simulink model "simulink"  (R2015a)
settings: Solver=ode4  StartTime=0.0  StopTime=inf  FixedStep=1e-3  RelTol=1e-3
values from neighbouring files (symbols this model uses):
  b_end1 = 0.5*(k_end1*Cyl1.m)^0.5    [m-script.m]
  b_end2 = 0.5*(k_end2*Cyl2.m)^0.5    [m-script.m]
  b_end3 = 0.5*(k_end3*Cyl3.m)^0.5    [m-script.m]
  b_end4 = 0.5*(k_end4*Cyl4.m)^0.5    [m-script.m]
  Cyl1_b = 40000    [m-script.m]
  Cyl1_Fc = 20514    [m-script.m]
  Cyl1_Fs = 22360    [m-script.m]
  Cyl1_K = 20000    [m-script.m]
  Cyl1_vs = 0.8    [m-script.m]
  Cyl2_b = 30000    [m-script.m]
  Cyl2_Fc = 14950    [m-script.m]
  Cyl2_Fs = 16125    [m-script.m]
  Cyl2_K = 20000    [m-script.m]
  Cyl2_vs = 0.8    [m-script.m]
  Cyl3_b = 30000    [m-script.m]
  Cyl3_Fc = 14996    [m-script.m]
  Cyl3_Fs = 16340    [m-script.m]
  Cyl3_K = 20000    [m-script.m]
  Cyl3_vs = 0.8    [m-script.m]
  Cyl4_b = 8500    [m-script.m]
  Cyl4_Fc = 4570    [m-script.m]
  Cyl4_Fs = 4945    [m-script.m]
  Cyl4_K = 20000    [m-script.m]
  Cyl4_vs = 0.8    [m-script.m]
  k_end1 = (pr_Ps*Cyl1.A_A)/v1    [m-script.m]
  k_end2 = (pr_Ps*Cyl2.A_A)/v2    [m-script.m]
  k_end3 = (pr_Ps*Cyl3.A_A)/v3    [m-script.m]
  k_end4 = (pr_Ps*Cyl4.A_A)/v4    [m-script.m]
  pr_Ps = 215e5    (= 21500000)    [m-script.m]
  sampleTime = 0.001    [m-script.m]
  Valve_eta = 0.989    [m-script.m]
  Valve_omega = 40.5    [m-script.m]
undefined symbols (not defined in the file or in its folder): Cyl, Cyl1, Cyl2, Cyl3, Cyl4, Cylinder2, Cylinder3, Cylinder4, Extention1, Extention2, Lift, Link1, Pillar, Pinion, Piston2, Piston3, Piston4, Rack, Tilt, Valve, X, Y, Z
undefined symbols (not defined in the file): Valve1, Valve2, Valve3, Valve4
libraries: sm_lib x72, simulink x32, nesl_utility x20, simulink_extras x3, xpcrtudplib x2, xpcobsoletelib x2
(part 3 of 4)

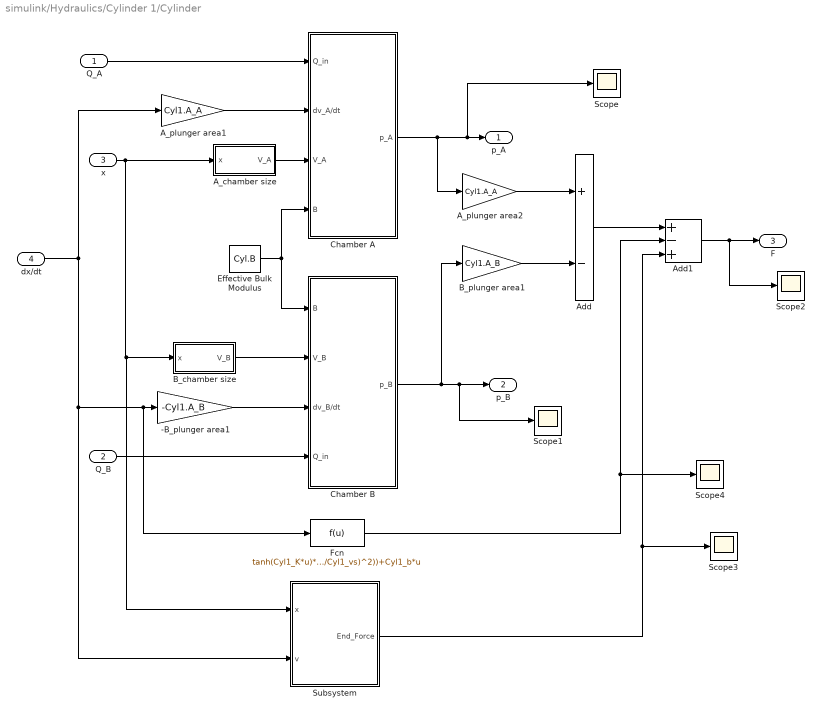
== system simulink/Hydraulics/Cylinder 1/Cylinder ==
  Q_A : Inport
  Q_B : Inport  Port=2
  x : Inport  Port=3
  dx/dt : Inport  Port=4
  -B_plunger area1 : Gain  Gain=-Cyl1.A_B
  A_chamber size : Subsystem
  A_plunger area1 : Gain  Gain=Cyl1.A_A
  A_plunger area2 : Gain  Gain=Cyl1.A_A
  Add : Sum  Inputs=+-
  Add1 : Sum  Inputs=+-+
  B_chamber size : Subsystem
  B_plunger area1 : Gain  Gain=Cyl1.A_B
  Chamber A : Subsystem  mask(Hydraulic){pinitial=Cyl1.pa_init}
      mask prompts: pinitial "Initial pressure [Pa] :"
      mask help: Lumped fluid volume. Pressure is limited greater or equal to zero by saturation block corresponding to a rough model of cavitation.
      mask Help: eval('hydlibdoc(''vol_cav_doc'')')
  Chamber B : Subsystem  mask(Hydraulic){pinitial=Cyl1.pb_init}
      mask prompts: pinitial "Initial pressure [Pa] :"
      mask help: Lumped fluid volume. Pressure is limited greater or equal to zero by saturation block corresponding to a rough model of cavitation.
      mask Help: eval('hydlibdoc(''vol_cav_doc'')')
  Effective Bulk Modulus : Constant  Value=Cyl.B
  Fcn : Fcn  Expr=tanh(Cyl1_K*u)*(Cyl1_Fc+(Cyl1_Fs-Cyl1_Fc)*exp(-1*(u/Cyl1_vs)^2))+Cyl1_b*u
  Scope{,1..4} (5 alike) : Scope
      Scope settings: YMin=4436994.34916  YMax=4451445.07232  SaveName=ScopeData34
      Scope1 settings: YMin=4437551.75654  YMax=4442034.19114  SaveName=ScopeData35
      Scope2 settings: YMin=-2641181.18354  YMax=577446.09906  SaveName=ScopeData5
      Scope3 settings: YMin=-2960719.83587  YMax=328968.87065  SaveName=ScopeData6
      Scope4 settings: YMin=-12307.20024  YMax=12364.555  SaveName=ScopeData7
  Subsystem : Subsystem
  p_A : Outport
  p_B : Outport  Port=2
  F : Outport  Port=3
  wires:
  A_plunger area1/1 -> Chamber A/2(" dv_A/dt")
  dx/dt/1 -> A_plunger area1/1, Subsystem/2(v), Fcn/1, -B_plunger area1/1
  Effective Bulk Modulus/1 -> Chamber A/4(" B"), Chamber B/1(B)
  -B_plunger area1/1 -> Chamber B/3(dv_B/dt)
  A_chamber size/1(V_A) -> Chamber A/3(" V_A")
  Fcn/1 -> Add1/2, Scope4/1
  Q_A/1 -> Chamber A/1(Q_in)
  Chamber A/1(p_A) -> Scope/1, p_A/1, A_plunger area2/1
  Chamber B/1(p_B) -> Scope1/1, p_B/1, B_plunger area1/1
  A_plunger area2/1 -> Add/1
  B_plunger area1/1 -> Add/2
  Add/1 -> Add1/1
  B_chamber size/1(V_B) -> Chamber B/2(V_B)
  Q_B/1 -> Chamber B/4(Q_in)
  Add1/1 -> Scope2/1, F/1
  x/1 -> A_chamber size/1(x), Subsystem/1(x), B_chamber size/1(x)
  Subsystem/1(End_Force) -> Add1/3, Scope3/1

== system simulink/Hydraulics/Cylinder 2/4//3 Valve ==
  p_A : Inport
  p_S : Inport  Port=2
  p_T : Inport  Port=3
  u : Inport  Port=4
  p_B : Inport  Port=5
  Flow paths : Subsystem
  Relative openings : Subsystem
  Valve Dynamics : Subsystem
  Q_P : Outport
  Q_T : Outport  Port=2
  Q_A : Outport  Port=3
  Q_B : Outport  Port=4
  wires:
  Valve Dynamics/1(x) -> Relative openings/1(x)
  Relative openings/1(av_AT) -> Flow paths/5(av_AT)
  Flow paths/4(Q_B) -> Q_B/1
  Flow paths/3(Q_T) -> Q_T/1
  Flow paths/2(Q_P) -> Q_P/1
  Flow paths/1(Q_A) -> Q_A/1
  p_T/1 -> Flow paths/4(p_T)
  p_S/1 -> Flow paths/3(p_S)
  p_B/1 -> Flow paths/2(p_B)
  p_A/1 -> Flow paths/1(p_A)
  Relative openings/2(av_BT) -> Flow paths/6(av_BT)
  Relative openings/3(av_PB) -> Flow paths/7(av_PB)
  Relative openings/4(av_PA) -> Flow paths/8(av_PA)
  u/1 -> Valve Dynamics/1(u)

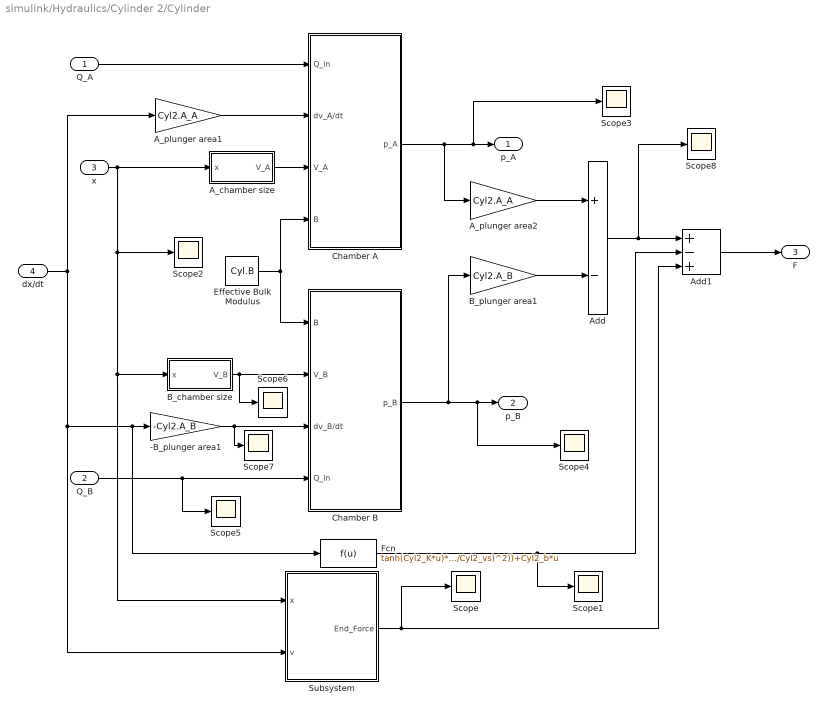
== system simulink/Hydraulics/Cylinder 2/Cylinder ==
  Q_A : Inport
  Q_B : Inport  Port=2
  x : Inport  Port=3
  dx/dt : Inport  Port=4
  -B_plunger area1 : Gain  Gain=-Cyl2.A_B
  A_chamber size : Subsystem
  A_plunger area1 : Gain  Gain=Cyl2.A_A
  A_plunger area2 : Gain  Gain=Cyl2.A_A
  Add : Sum  Inputs=+-
  Add1 : Sum  Inputs=+-+
  B_chamber size : Subsystem
  B_plunger area1 : Gain  Gain=Cyl2.A_B
  Chamber A : Subsystem  mask(Hydraulic){pinitial=Cyl2.pa_init}
      mask prompts: pinitial "Initial pressure [Pa] :"
      mask help: Lumped fluid volume. Pressure is limited greater or equal to zero by saturation block corresponding to a rough model of cavitation.
      mask Help: eval('hydlibdoc(''vol_cav_doc'')')
  Chamber B : Subsystem  mask(Hydraulic){pinitial=Cyl2.pb_init}
      mask prompts: pinitial "Initial pressure [Pa] :"
      mask help: Lumped fluid volume. Pressure is limited greater or equal to zero by saturation block corresponding to a rough model of cavitation.
      mask Help: eval('hydlibdoc(''vol_cav_doc'')')
  Effective Bulk Modulus : Constant  Value=Cyl.B
  Fcn : Fcn  Expr=tanh(Cyl2_K*u)*(Cyl2_Fc+(Cyl2_Fs-Cyl2_Fc)*exp(-1*(u/Cyl2_vs)^2))+Cyl2_b*u
  Scope{,1..8} (9 alike) : Scope
      Scope settings: YMin=-1051842.78204  YMax=116871.42023  SaveName=ScopeData2
      Scope1 settings: YMin=-10637.267  YMax=10226.6678  SaveName=ScopeData4
      Scope2 settings: YMin=0.22817  YMax=0.24759  SaveName=ScopeData5
      Scope3 settings: YMin=10697580.90994  YMax=17121771.81053  SaveName=ScopeData32
      Scope4 settings: YMin=1984662.3633  YMax=2265607.51831  SaveName=ScopeData33
      Scope5 settings: YMin=-0.00000009  YMax=0.00000026
      Scope6 settings: YMin=-0.00041  YMax=0.00539  SaveName=ScopeData2
      Scope7 settings: YMin=-0.00176  YMax=0.00311  SaveName=ScopeData7
      Scope8 settings: YMin=79251.57966  YMax=181198.26244  SaveName=ScopeData2
  Subsystem : Subsystem
  p_A : Outport
  p_B : Outport  Port=2
  F : Outport  Port=3
  wires:
  A_plunger area1/1 -> Chamber A/2(" dv_A/dt")
  dx/dt/1 -> A_plunger area1/1, Fcn/1, -B_plunger area1/1, Subsystem/2(v)
  Effective Bulk Modulus/1 -> Chamber A/4(" B"), Chamber B/1(B)
  x/1 -> A_chamber size/1(x), Scope2/1, Subsystem/1(x), B_chamber size/1(x)
  -B_plunger area1/1 -> Scope7/1, Chamber B/3(dv_B/dt)
  A_chamber size/1(V_A) -> Chamber A/3(" V_A")
  Fcn/1 -> Scope1/1, Add1/2
  Q_A/1 -> Chamber A/1(Q_in)
  Chamber A/1(p_A) -> Scope3/1, p_A/1, A_plunger area2/1
  Chamber B/1(p_B) -> Scope4/1, p_B/1, B_plunger area1/1
  A_plunger area2/1 -> Add/1
  B_plunger area1/1 -> Add/2
  Add/1 -> Scope8/1, Add1/1
  B_chamber size/1(V_B) -> Chamber B/2(V_B), Scope6/1
  Q_B/1 -> Scope5/1, Chamber B/4(Q_in)
  Add1/1 -> F/1
  Subsystem/1(End_Force) -> Scope/1, Add1/3

== system simulink/Hydraulics/Cylinder 3/4//3 Valve ==
  p_A : Inport
  p_S : Inport  Port=2
  p_T : Inport  Port=3
  u : Inport  Port=4
  p_B : Inport  Port=5
  Flow paths : Subsystem
  Relative openings : Subsystem
  Valve Dynamics : Subsystem
  Q_P : Outport
  Q_T : Outport  Port=2
  Q_A : Outport  Port=3
  Q_B : Outport  Port=4
  wires:
  Valve Dynamics/1(x) -> Relative openings/1(x)
  Relative openings/1(av_AT) -> Flow paths/5(av_AT)
  Flow paths/4(Q_B) -> Q_B/1
  Flow paths/3(Q_T) -> Q_T/1
  Flow paths/2(Q_P) -> Q_P/1
  Flow paths/1(Q_A) -> Q_A/1
  p_T/1 -> Flow paths/4(p_T)
  p_S/1 -> Flow paths/3(p_S)
  p_B/1 -> Flow paths/2(p_B)
  p_A/1 -> Flow paths/1(p_A)
  Relative openings/2(av_BT) -> Flow paths/6(av_BT)
  Relative openings/3(av_PB) -> Flow paths/7(av_PB)
  Relative openings/4(av_PA) -> Flow paths/8(av_PA)
  u/1 -> Valve Dynamics/1(u)

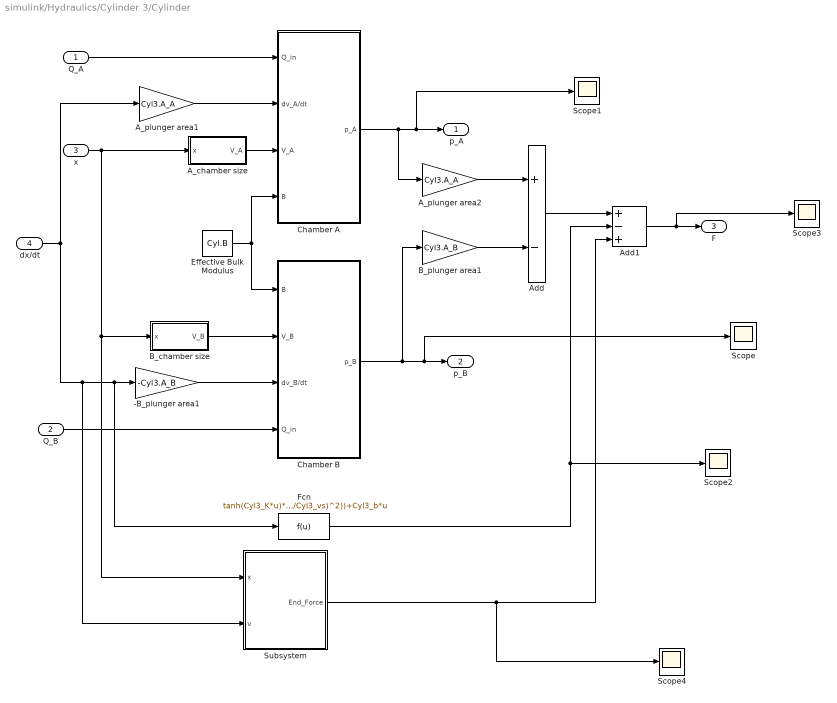
== system simulink/Hydraulics/Cylinder 3/Cylinder ==
  Q_A : Inport
  Q_B : Inport  Port=2
  x : Inport  Port=3
  dx/dt : Inport  Port=4
  -B_plunger area1 : Gain  Gain=-Cyl3.A_B
  A_chamber size : Subsystem
  A_plunger area1 : Gain  Gain=Cyl3.A_A
  A_plunger area2 : Gain  Gain=Cyl3.A_A
  Add : Sum  Inputs=+-
  Add1 : Sum  Inputs=+-+
  B_chamber size : Subsystem
  B_plunger area1 : Gain  Gain=Cyl3.A_B
  Chamber A : Subsystem  mask(Hydraulic){pinitial=Cyl3.pa_init}
      mask prompts: pinitial "Initial pressure [Pa] :"
      mask help: Lumped fluid volume. Pressure is limited greater or equal to zero by saturation block corresponding to a rough model of cavitation.
      mask Help: eval('hydlibdoc(''vol_cav_doc'')')
  Chamber B : Subsystem  mask(Hydraulic){pinitial=Cyl3.pb_init}
      mask prompts: pinitial "Initial pressure [Pa] :"
      mask help: Lumped fluid volume. Pressure is limited greater or equal to zero by saturation block corresponding to a rough model of cavitation.
      mask Help: eval('hydlibdoc(''vol_cav_doc'')')
  Effective Bulk Modulus : Constant  Value=Cyl.B
  Fcn : Fcn  Expr=tanh(Cyl3_K*u)*(Cyl3_Fc+(Cyl3_Fs-Cyl3_Fc)*exp(-1*(u/Cyl3_vs)^2))+Cyl3_b*u
  Scope{,1..4} (5 alike) : Scope
      Scope settings: YMin=-232506.13833  YMax=2092555.24493  SaveName=ScopeData30
      Scope1 settings: YMin=8204020.85918  YMax=9658590.83811  SaveName=ScopeData31
      Scope2 settings: YMin=-10  YMax=10  SaveName=ScopeData2
      Scope3 settings: YMin=-10  YMax=10  SaveName=ScopeData3
      Scope4 settings: YMin=-453635.79942  YMax=50403.97771  SaveName=ScopeData4
  Subsystem : Subsystem
  p_A : Outport
  p_B : Outport  Port=2
  F : Outport  Port=3
  wires:
  A_plunger area1/1 -> Chamber A/2(" dv_A/dt")
  dx/dt/1 -> A_plunger area1/1, Subsystem/2(v), -B_plunger area1/1, Fcn/1
  Effective Bulk Modulus/1 -> Chamber A/4(" B"), Chamber B/1(B)
  x/1 -> A_chamber size/1(x), Subsystem/1(x), B_chamber size/1(x)
  -B_plunger area1/1 -> Chamber B/3(dv_B/dt)
  A_chamber size/1(V_A) -> Chamber A/3(" V_A")
  Fcn/1 -> Scope2/1, Add1/2
  Q_A/1 -> Chamber A/1(Q_in)
  Chamber A/1(p_A) -> Scope1/1, p_A/1, A_plunger area2/1
  Chamber B/1(p_B) -> Scope/1, p_B/1, B_plunger area1/1
  A_plunger area2/1 -> Add/1
  B_plunger area1/1 -> Add/2
  Add/1 -> Add1/1
  B_chamber size/1(V_B) -> Chamber B/2(V_B)
  Q_B/1 -> Chamber B/4(Q_in)
  Subsystem/1(End_Force) -> Scope4/1, Add1/3
  Add1/1 -> Scope3/1, F/1

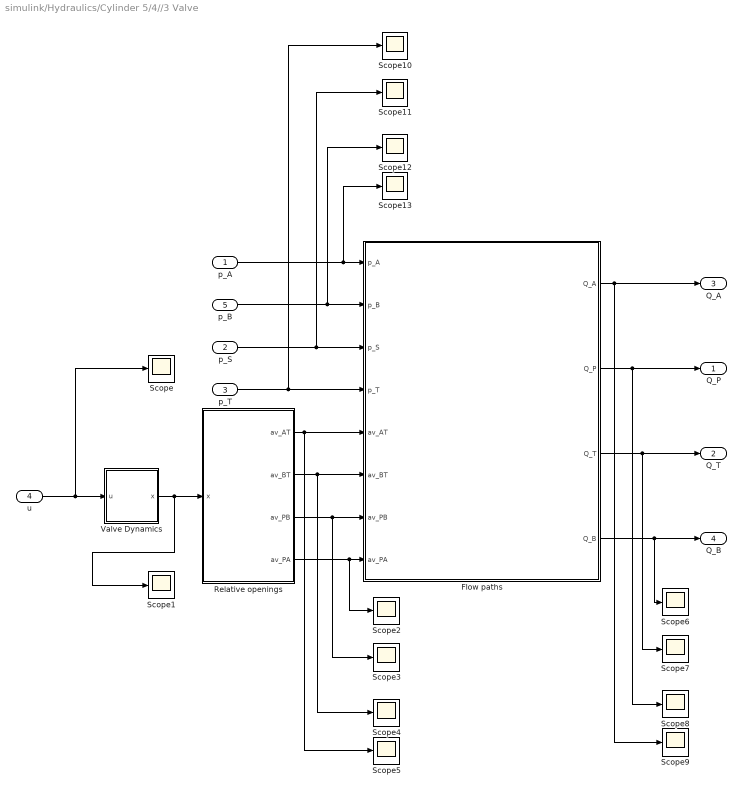
== system simulink/Hydraulics/Cylinder 5/4//3 Valve ==
  p_A : Inport
  p_S : Inport  Port=2
  p_T : Inport  Port=3
  u : Inport  Port=4
  p_B : Inport  Port=5
  Flow paths : Subsystem
  Relative openings : Subsystem
  Scope{,1..13} (14 alike) : Scope
      Scope settings: YMin=-1.00000  YMax=1.00000  SaveName=ScopeData9
      Scope1 settings: YMin=0.1317  YMax=0.45561  SaveName=ScopeData10
      Scope10 settings: YMin=-1.00000  YMax=1.00000  SaveName=ScopeData19
      Scope11 settings: YMin=11500000.00000  YMax=31500000.00000  SaveName=ScopeData20
      Scope12 settings: YMin=-2997924.65507  YMax=26981321.89563  SaveName=ScopeData21
      Scope13 settings: YMin=-2854848.69891  YMax=25693638.29022  SaveName=ScopeData22
      Scope2 settings: YMin=0.00049  YMax=0.00069  SaveName=ScopeData11
      Scope3 settings: YMin=0.00049  YMax=0.00069  SaveName=ScopeData12
      Scope4 settings: YMin=0.00015  YMax=0.00215  SaveName=ScopeData13
      Scope5 settings: YMin=0.00015  YMax=0.00215  SaveName=ScopeData14
      Scope6 settings: YMin=-0.00461  YMax=0.00297  SaveName=ScopeData15
      Scope7 settings: YMin=0.0000081  YMax=0.0000153  SaveName=ScopeData16
      Scope8 settings: YMin=-0.0000093  YMax=-0.000006  SaveName=ScopeData17
      Scope9 settings: YMin=-0.000009  YMax=0.000001  SaveName=ScopeData18
  Valve Dynamics : Subsystem
  Q_P : Outport
  Q_T : Outport  Port=2
  Q_A : Outport  Port=3
  Q_B : Outport  Port=4
  wires:
  u/1 -> Scope/1, Valve Dynamics/1(u)
  Relative openings/3(av_PB) -> Scope3/1, Flow paths/7(av_PB)
  Relative openings/2(av_BT) -> Scope4/1, Flow paths/6(av_BT)
  p_A/1 -> Scope13/1, Flow paths/1(p_A)
  p_B/1 -> Scope12/1, Flow paths/2(p_B)
  p_S/1 -> Scope11/1, Flow paths/3(p_S)
  p_T/1 -> Scope10/1, Flow paths/4(p_T)
  Flow paths/1(Q_A) -> Scope9/1, Q_A/1
  Flow paths/2(Q_P) -> Scope8/1, Q_P/1
  Flow paths/3(Q_T) -> Scope7/1, Q_T/1
  Flow paths/4(Q_B) -> Scope6/1, Q_B/1
  Relative openings/1(av_AT) -> Scope5/1, Flow paths/5(av_AT)
  Valve Dynamics/1(x) -> Scope1/1, Relative openings/1(x)
  Relative openings/4(av_PA) -> Scope2/1, Flow paths/8(av_PA)

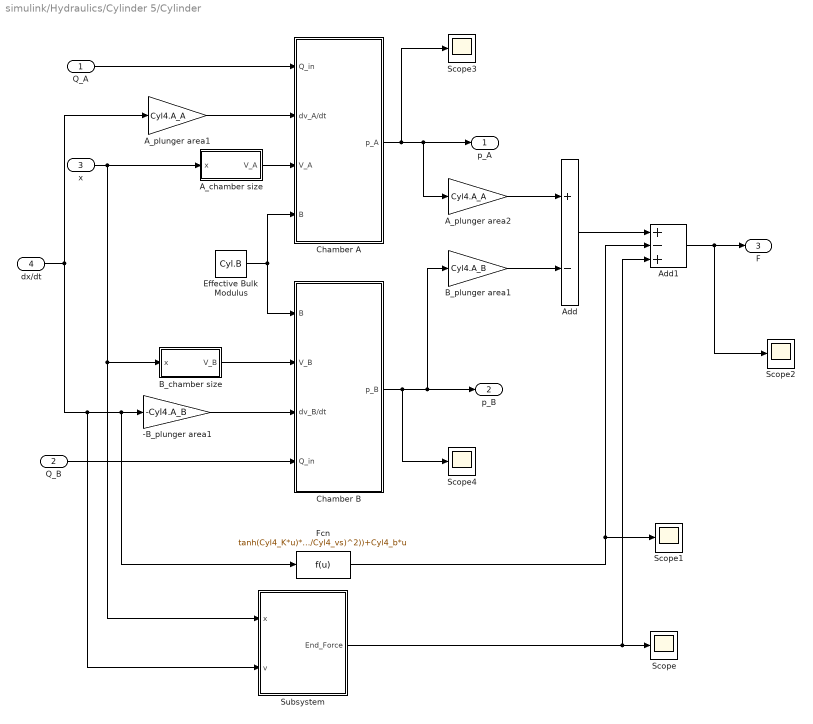
== system simulink/Hydraulics/Cylinder 5/Cylinder ==
  Q_A : Inport
  Q_B : Inport  Port=2
  x : Inport  Port=3
  dx/dt : Inport  Port=4
  -B_plunger area1 : Gain  Gain=-Cyl4.A_B
  A_chamber size : Subsystem
  A_plunger area1 : Gain  Gain=Cyl4.A_A
  A_plunger area2 : Gain  Gain=Cyl4.A_A
  Add : Sum  Inputs=+-
  Add1 : Sum  Inputs=+-+
  B_chamber size : Subsystem
  B_plunger area1 : Gain  Gain=Cyl4.A_B
  Chamber A : Subsystem  mask(Hydraulic){pinitial=Cyl4.pa_init}
      mask prompts: pinitial "Initial pressure [Pa] :"
      mask help: Lumped fluid volume. Pressure is limited greater or equal to zero by saturation block corresponding to a rough model of cavitation.
      mask Help: eval('hydlibdoc(''vol_cav_doc'')')
  Chamber B : Subsystem  mask(Hydraulic){pinitial=Cyl4.pb_init}
      mask prompts: pinitial "Initial pressure [Pa] :"
      mask help: Lumped fluid volume. Pressure is limited greater or equal to zero by saturation block corresponding to a rough model of cavitation.
      mask Help: eval('hydlibdoc(''vol_cav_doc'')')
  Effective Bulk Modulus : Constant  Value=Cyl.B
  Fcn : Fcn  Expr=tanh(Cyl4_K*u)*(Cyl4_Fc+(Cyl4_Fs-Cyl4_Fc)*exp(-1*(u/Cyl4_vs)^2))+Cyl4_b*u
  Scope{,1..4} (5 alike) : Scope
      Scope settings: YMin=-102297.75524  YMax=11366.41725
      Scope1 settings: YMin=-7398.06306  YMax=8052.93154  SaveName=ScopeData2
      Scope2 settings: YMin=-14569.30146  YMax=3367.51691  SaveName=ScopeData3
      Scope3 settings: YMin=2510985.33452  YMax=2517001.5388  SaveName=ScopeData23
      Scope4 settings: YMin=-3100765.75474  YMax=27906891.79262  SaveName=ScopeData24
  Subsystem : Subsystem
  p_A : Outport
  p_B : Outport  Port=2
  F : Outport  Port=3
  wires:
  Subsystem/1(End_Force) -> Scope/1, Add1/3
  Add1/1 -> Scope2/1, F/1
  Q_B/1 -> Chamber B/4(Q_in)
  B_chamber size/1(V_B) -> Chamber B/2(V_B)
  Add/1 -> Add1/1
  B_plunger area1/1 -> Add/2
  A_plunger area2/1 -> Add/1
  Chamber B/1(p_B) -> Scope4/1, B_plunger area1/1, p_B/1
  Chamber A/1(p_A) -> Scope3/1, A_plunger area2/1, p_A/1
  Q_A/1 -> Chamber A/1(Q_in)
  Fcn/1 -> Scope1/1, Add1/2
  A_chamber size/1(V_A) -> Chamber A/3(" V_A")
  -B_plunger area1/1 -> Chamber B/3(dv_B/dt)
  x/1 -> B_chamber size/1(x), Subsystem/1(x), A_chamber size/1(x)
  Effective Bulk Modulus/1 -> Chamber B/1(B), Chamber A/4(" B")
  dx/dt/1 -> Fcn/1, -B_plunger area1/1, Subsystem/2(v), A_plunger area1/1
  A_plunger area1/1 -> Chamber A/2(" dv_A/dt")

== system simulink/Hydraulics/Cylinder 1/4//3 Valve/Flow paths ==
  p_A : Inport
  p_B : Inport  Port=2
  p_S : Inport  Port=3
  p_T : Inport  Port=4
  av_AT : Inport  Port=5
  av_BT : Inport  Port=6
  av_PB : Inport  Port=7
  av_PA : Inport  Port=8
  Orifice AT : Subsystem  mask(Hydraulic){QN=Valve1.QN.AT, dpN=Valve1.dpN, ptr=Valve1.ptr}
      mask prompts: QN "Nominal Flow [m^3/s] :"; dpN "Nominal Pressure Difference [Pa] :"; ptr "Transition Pressure [Pa] :"
      mask help:
      | Implements numerically robust turbulent flow
      | equation. Polynomial flow equation is used
      | when abs(dp) < Transition Pressure.
      mask init:
      | K = QN/(sqrt(dpN));
      mask Help: eval('hydlibdoc(''orificedoc'')')
  Orifice BT : Subsystem  mask(Hydraulic){QN=Valve1.QN.BT, dpN=Valve1.dpN, ptr=Valve1.ptr}
      mask prompts: QN "Nominal Flow [m^3/s] :"; dpN "Nominal Pressure Difference [Pa] :"; ptr "Transition Pressure [Pa] :"
      mask help:
      | Implements numerically robust turbulent flow
      | equation. Polynomial flow equation is used
      | when abs(dp) < Transition Pressure.
      mask init:
      | K = QN/(sqrt(dpN));
      mask Help: eval('hydlibdoc(''orificedoc'')')
  Orifice PA : Subsystem  mask(Hydraulic){QN=Valve1.QN.PA, dpN=Valve1.dpN, ptr=Valve1.ptr}
      mask prompts: QN "Nominal Flow [m^3/s] :"; dpN "Nominal Pressure Difference [Pa] :"; ptr "Transition Pressure [Pa] :"
      mask help:
      | Implements numerically robust turbulent flow
      | equation. Polynomial flow equation is used
      | when abs(dp) < Transition Pressure.
      mask init:
      | K = QN/(sqrt(dpN));
      mask Help: eval('hydlibdoc(''orificedoc'')')
  Orifice PB : Subsystem  mask(Hydraulic){QN=Valve1.QN.PB, dpN=Valve1.dpN, ptr=Valve1.ptr}
      mask prompts: QN "Nominal Flow [m^3/s] :"; dpN "Nominal Pressure Difference [Pa] :"; ptr "Transition Pressure [Pa] :"
      mask help:
      | Implements numerically robust turbulent flow
      | equation. Polynomial flow equation is used
      | when abs(dp) < Transition Pressure.
      mask init:
      | K = QN/(sqrt(dpN));
      mask Help: eval('hydlibdoc(''orificedoc'')')
  Sum{,1..3} (4 alike) : Sum  Inputs=|++
  Q_A : Outport
  Q_P : Outport  Port=2
  Q_T : Outport  Port=3
  Q_B : Outport  Port=4
  wires:
  p_A/1 -> Orifice AT/1(p_A), Orifice PA/2(p_A)
  p_T/1 -> Orifice BT/1(p_T), Orifice AT/2(p_T)
  av_BT/1 -> Orifice BT/3(u)
  av_PA/1 -> Orifice PA/3(u)
  p_B/1 -> Orifice PB/1(p_B), Orifice BT/2(p_B)
  av_PB/1 -> Orifice PB/3(u)
  p_S/1 -> Orifice PB/2(p_P), Orifice PA/1(p_P)
  av_AT/1 -> Orifice AT/3(u)
  Orifice PA/2(Q_A) -> Sum/1
  Orifice AT/1(Q_A) -> Sum/2
  Orifice AT/2(Q_T) -> Sum3/1
  Orifice BT/1(Q_T) -> Sum3/2
  Orifice BT/2(Q_B) -> Sum2/1
  Orifice PB/1(Q_B) -> Sum2/2
  Orifice PA/1(Q_P) -> Sum1/1
  Orifice PB/2(Q_P) -> Sum1/2
  Sum/1 -> Q_A/1
  Sum1/1 -> Q_P/1
  Sum3/1 -> Q_T/1
  Sum2/1 -> Q_B/1

== system simulink/Hydraulics/Cylinder 1/4//3 Valve/Relative openings ==
  x : Inport
  Lookup Table AT : Lookup_n-D  NumberOfTableDimensions=1  BreakpointsForDimension1=Valve.lookupspoolAT  Table=Valve.lookupopenAT  InternalRulePriority=Speed  RndMeth=Simplest  InputSameDT=on
  Lookup Table BT : Lookup_n-D  NumberOfTableDimensions=1  BreakpointsForDimension1=Valve.lookupspoolBT  Table=Valve.lookupopenBT  InternalRulePriority=Speed  RndMeth=Simplest  InputSameDT=on
  Lookup Table PA : Lookup_n-D  NumberOfTableDimensions=1  BreakpointsForDimension1=Valve.lookupspoolPA  Table=Valve.lookupopenPA  InternalRulePriority=Speed  RndMeth=Simplest  InputSameDT=on
  Lookup Table PB : Lookup_n-D  NumberOfTableDimensions=1  BreakpointsForDimension1=Valve.lookupspoolPB  Table=Valve.lookupopenPB  InternalRulePriority=Speed  RndMeth=Simplest  InputSameDT=on
  av_AT : Outport
  av_BT : Outport  Port=2
  av_PB : Outport  Port=3
  av_PA : Outport  Port=4
  wires:
  x/1 -> Lookup Table AT/1, Lookup Table PB/1, Lookup Table BT/1, Lookup Table PA/1
  Lookup Table AT/1 -> av_AT/1
  Lookup Table PA/1 -> av_PA/1
  Lookup Table BT/1 -> av_BT/1
  Lookup Table PB/1 -> av_PB/1

== system simulink/Hydraulics/Cylinder 1/4//3 Valve/Valve Dynamics ==
  u : Inport
  Saturation1 : Saturate  UpperLimit=1  LowerLimit=-1
  Transfer Fcn1 : TransferFcn  Numerator=[(Valve_omega)^2]  Denominator=[1 2*Valve_eta*Valve_omega (Valve_omega)^2]
  Transport Delay1 : TransportDelay  DelayTime=Valve.secondorder_delay
  x : Outport
  wires:
  Transfer Fcn1/1 -> Saturation1/1
  u/1 -> Transport Delay1/1
  Saturation1/1 -> x/1
  Transport Delay1/1 -> Transfer Fcn1/1

== system simulink/Hydraulics/Cylinder 1/Cylinder/A_chamber size ==
  x : Inport
  A_Dead Vol : Constant  Value=Cyl.V0A
  A_plunger area : Gain  Gain=Cyl1.A_A
  Add1 : Sum
  V_A : Outport
  wires:
  A_Dead Vol/1 -> Add1/2
  A_plunger area/1 -> Add1/1
  x/1 -> A_plunger area/1
  Add1/1 -> V_A/1

== system simulink/Hydraulics/Cylinder 1/Cylinder/B_chamber size ==
  x : Inport
  Add2 : Sum  Inputs=-+
  Add4 : Sum
  B_Dead Vol : Constant  Value=Cyl.V0B
  B_plunger area : Gain  Gain=Cyl1.A_B
  Cyl_stroke : Constant  Value=Cyl1.xmax
  V_B : Outport
  wires:
  Add4/1 -> V_B/1
  B_Dead Vol/1 -> Add4/2
  B_plunger area/1 -> Add4/1
  Add2/1 -> B_plunger area/1
  x/1 -> Add2/1
  Cyl_stroke/1 -> Add2/2

== system simulink/Hydraulics/Cylinder 1/Cylinder/Chamber A ==
  Q_in : Inport
  " dv_A/dt" : Inport  Port=2
  " V_A" : Inport  Port=3
  " B" : Inport  Port=4
  Integrator : Integrator  InitialCondition=pinitial  AbsoluteTolerance=10
  Product : Product  Inputs=*/*  SaturateOnIntegerOverflow=on  InputSameDT=on  OutDataTypeStr=Inherit: Same as first input
  Saturation : Saturate  UpperLimit=inf  LowerLimit=0
  Sum : Sum  Inputs=+-  SaturateOnIntegerOverflow=on  InputSameDT=on  OutDataTypeStr=Inherit: Same as first input
  p_A : Outport
  wires:
  Sum/1 -> Product/1
  Q_in/1 -> Sum/1
  " B"/1 -> Product/3
  Saturation/1 -> p_A/1
  Integrator/1 -> Saturation/1
  Product/1 -> Integrator/1
  " dv_A/dt"/1 -> Sum/2
  " V_A"/1 -> Product/2

== system simulink/Hydraulics/Cylinder 1/Cylinder/Chamber B ==
  B : Inport
  V_B : Inport  Port=2
  dv_B/dt : Inport  Port=3
  Q_in : Inport  Port=4
  Integrator : Integrator  InitialCondition=pinitial  AbsoluteTolerance=10
  Product : Product  Inputs=*/*  SaturateOnIntegerOverflow=on  InputSameDT=on  OutDataTypeStr=Inherit: Same as first input
  Saturation : Saturate  UpperLimit=inf  LowerLimit=0
  Sum : Sum  Inputs=+-  SaturateOnIntegerOverflow=on  InputSameDT=on  OutDataTypeStr=Inherit: Same as first input
  p_B : Outport
  wires:
  Product/1 -> Integrator/1
  Integrator/1 -> Saturation/1
  Saturation/1 -> p_B/1
  B/1 -> Product/3
  Q_in/1 -> Sum/1
  Sum/1 -> Product/1
  dv_B/dt/1 -> Sum/2
  V_B/1 -> Product/2

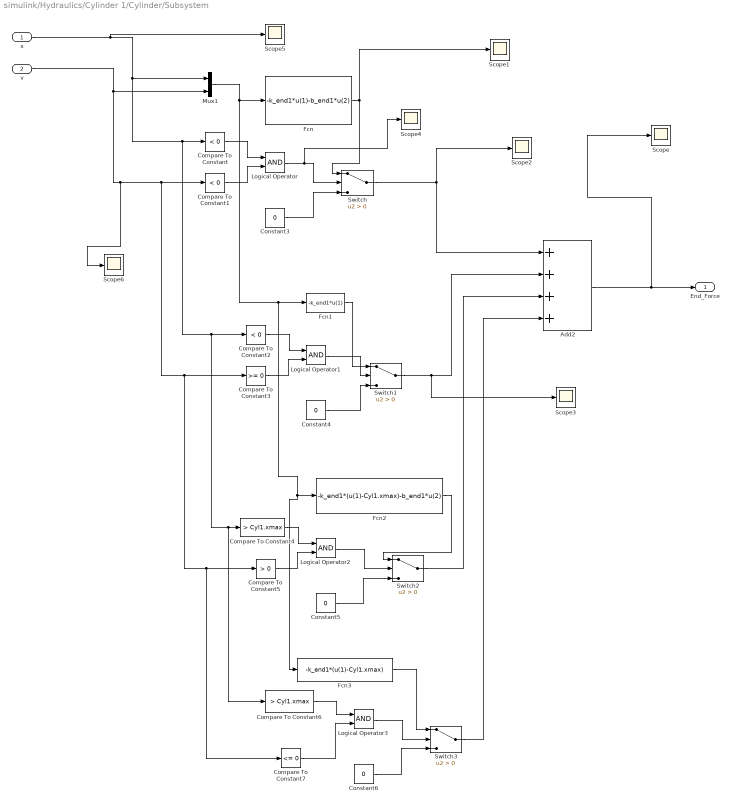
== system simulink/Hydraulics/Cylinder 1/Cylinder/Subsystem ==
  x : Inport
  v : Inport  Port=2
  Add2 : Sum  Inputs=++++
  Compare To Constant : simulink/Logic and Bit Operations/Compare To Constant  relop=<  const=0  OutDataTypeStr=boolean
  Compare To Constant1 : simulink/Logic and Bit Operations/Compare To Constant  relop=<  const=0  OutDataTypeStr=boolean
  Compare To Constant2 : simulink/Logic and Bit Operations/Compare To Constant  relop=<  const=0  OutDataTypeStr=boolean
  Compare To Constant3 : simulink/Logic and Bit Operations/Compare To Constant  relop=>=  const=0  OutDataTypeStr=boolean
  Compare To Constant4 : simulink/Logic and Bit Operations/Compare To Constant  relop=>  const=Cyl1.xmax  OutDataTypeStr=boolean
  Compare To Constant5 : simulink/Logic and Bit Operations/Compare To Constant  relop=>  const=0  OutDataTypeStr=boolean
  Compare To Constant6 : simulink/Logic and Bit Operations/Compare To Constant  relop=>  const=Cyl1.xmax  OutDataTypeStr=boolean
  Compare To Constant7 : simulink/Logic and Bit Operations/Compare To Constant  relop=<=  const=0  OutDataTypeStr=boolean
  Constant{3..6} (4 alike) : Constant  Value=0
  Fcn : Fcn  Expr=-k_end1*u(1)-b_end1*u(2)
  Fcn1 : Fcn  Expr=-k_end1*u(1)
  Fcn2 : Fcn  Expr=-k_end1*(u(1)-Cyl1.xmax)-b_end1*u(2)
  Fcn3 : Fcn  Expr=-k_end1*(u(1)-Cyl1.xmax)
  Logical Operator{,1..3} (4 alike) : Logic  AllPortsSameDT=off  OutDataTypeStr=boolean
  Mux1 : Mux  Inputs=2
  Scope{,1..6} (7 alike) : Scope
      Scope settings: YMin=-1.00000  YMax=1.00000  SaveName=ScopeData7
      Scope1 settings: YMin=-1321864731.63954  YMax=-746398119.03494  SaveName=ScopeData8
      Scope2 settings: YMin=-1.00000  YMax=1.00000  SaveName=ScopeData9
      Scope3 settings: YMin=-1626189.56555  YMax=14635706.08996  SaveName=ScopeData10
      Scope4 settings: YMin=-1.00000  YMax=1.00000  SaveName=ScopeData11
      Scope5 settings: YMin=0.45891  YMax=0.49078  SaveName=ScopeData12
      Scope6 settings: YMin=-0.00619  YMax=0.05469  SaveName=ScopeData13
  Switch{,1..3} (4 alike) : Switch  Criteria=u2 > Threshold
  End_Force : Outport
  wires:
  Compare To Constant3/1 -> Logical Operator1/2
  Fcn1/1 -> Switch1/1
  Compare To Constant4/1 -> Logical Operator2/1
  Compare To Constant/1 -> Logical Operator/1
  Constant3/1 -> Switch/3
  Logical Operator/1 -> Scope4/1, Switch/2
  Fcn/1 -> Switch/1, Scope1/1
  Logical Operator1/1 -> Switch1/2
  Constant4/1 -> Switch1/3
  Constant5/1 -> Switch2/3
  Compare To Constant1/1 -> Logical Operator/2
  Compare To Constant2/1 -> Logical Operator1/1
  Switch3/1 -> Add2/4
  Mux1/1 -> Fcn/1, Fcn3/1, Fcn2/1, Fcn1/1
  Add2/1 -> Scope/1, End_Force/1
  Switch1/1 -> Scope3/1, Add2/2
  Compare To Constant7/1 -> Logical Operator3/2
  Logical Operator2/1 -> Switch2/2
  Switch/1 -> Scope2/1, Add2/1
  Compare To Constant6/1 -> Logical Operator3/1
  Switch2/1 -> Add2/3
  Constant6/1 -> Switch3/3
  Compare To Constant5/1 -> Logical Operator2/2
  Fcn3/1 -> Switch3/1
  Logical Operator3/1 -> Switch3/2
  Fcn2/1 -> Switch2/1
  v/1 -> Scope6/1, Compare To Constant7/1, Compare To Constant5/1, Compare To Constant3/1, Compare To Constant1/1, Mux1/2
  x/1 -> Scope5/1, Mux1/1, Compare To Constant4/1, Compare To Constant6/1, Compare To Constant2/1, Compare To Constant/1

== system simulink/Hydraulics/Cylinder 2/4//3 Valve/Flow paths ==
  p_A : Inport
  p_B : Inport  Port=2
  p_S : Inport  Port=3
  p_T : Inport  Port=4
  av_AT : Inport  Port=5
  av_BT : Inport  Port=6
  av_PB : Inport  Port=7
  av_PA : Inport  Port=8
  Orifice AT : Subsystem  mask(Hydraulic){QN=Valve2.QN.AT, dpN=Valve2.dpN, ptr=Valve2.ptr}
      mask prompts: QN "Nominal Flow [m^3/s] :"; dpN "Nominal Pressure Difference [Pa] :"; ptr "Transition Pressure [Pa] :"
      mask help:
      | Implements numerically robust turbulent flow
      | equation. Polynomial flow equation is used
      | when abs(dp) < Transition Pressure.
      mask init:
      | K = QN/(sqrt(dpN));
      mask Help: eval('hydlibdoc(''orificedoc'')')
  Orifice BT : Subsystem  mask(Hydraulic){QN=Valve2.QN.BT, dpN=Valve2.dpN, ptr=Valve2.ptr}
      mask prompts: QN "Nominal Flow [m^3/s] :"; dpN "Nominal Pressure Difference [Pa] :"; ptr "Transition Pressure [Pa] :"
      mask help:
      | Implements numerically robust turbulent flow
      | equation. Polynomial flow equation is used
      | when abs(dp) < Transition Pressure.
      mask init:
      | K = QN/(sqrt(dpN));
      mask Help: eval('hydlibdoc(''orificedoc'')')
  Orifice PA : Subsystem  mask(Hydraulic){QN=Valve2.QN.PA, dpN=Valve2.dpN, ptr=Valve2.ptr}
      mask prompts: QN "Nominal Flow [m^3/s] :"; dpN "Nominal Pressure Difference [Pa] :"; ptr "Transition Pressure [Pa] :"
      mask help:
      | Implements numerically robust turbulent flow
      | equation. Polynomial flow equation is used
      | when abs(dp) < Transition Pressure.
      mask init:
      | K = QN/(sqrt(dpN));
      mask Help: eval('hydlibdoc(''orificedoc'')')
  Orifice PB : Subsystem  mask(Hydraulic){QN=Valve2.QN.PB, dpN=Valve2.dpN, ptr=Valve2.ptr}
      mask prompts: QN "Nominal Flow [m^3/s] :"; dpN "Nominal Pressure Difference [Pa] :"; ptr "Transition Pressure [Pa] :"
      mask help:
      | Implements numerically robust turbulent flow
      | equation. Polynomial flow equation is used
      | when abs(dp) < Transition Pressure.
      mask init:
      | K = QN/(sqrt(dpN));
      mask Help: eval('hydlibdoc(''orificedoc'')')
  Scope : Scope
      settings: YMin=-0.00424  YMax=0.00506  SaveName=ScopeData3
  Sum{,1..3} (4 alike) : Sum  Inputs=|++
  Q_A : Outport
  Q_P : Outport  Port=2
  Q_T : Outport  Port=3
  Q_B : Outport  Port=4
  wires:
  p_A/1 -> Orifice AT/1(p_A), Orifice PA/2(p_A)
  p_T/1 -> Orifice BT/1(p_T), Orifice AT/2(p_T)
  av_BT/1 -> Orifice BT/3(u)
  av_PA/1 -> Orifice PA/3(u)
  p_B/1 -> Orifice PB/1(p_B), Orifice BT/2(p_B)
  av_PB/1 -> Orifice PB/3(u)
  p_S/1 -> Orifice PB/2(p_P), Orifice PA/1(p_P)
  av_AT/1 -> Orifice AT/3(u)
  Orifice PA/2(Q_A) -> Sum/1
  Orifice AT/1(Q_A) -> Sum/2
  Orifice AT/2(Q_T) -> Sum3/1
  Orifice BT/1(Q_T) -> Sum3/2
  Orifice BT/2(Q_B) -> Sum2/1
  Orifice PB/1(Q_B) -> Sum2/2
  Orifice PA/1(Q_P) -> Sum1/1
  Orifice PB/2(Q_P) -> Sum1/2
  Sum/1 -> Q_A/1
  Sum1/1 -> Q_P/1
  Sum3/1 -> Q_T/1
  Sum2/1 -> Scope/1, Q_B/1

== system simulink/Hydraulics/Cylinder 2/4//3 Valve/Relative openings ==
  x : Inport
  Lookup Table AT : Lookup_n-D  NumberOfTableDimensions=1  BreakpointsForDimension1=Valve.lookupspoolAT  Table=Valve.lookupopenAT  InternalRulePriority=Speed  RndMeth=Simplest  InputSameDT=on
  Lookup Table BT : Lookup_n-D  NumberOfTableDimensions=1  BreakpointsForDimension1=Valve.lookupspoolBT  Table=Valve.lookupopenBT  InternalRulePriority=Speed  RndMeth=Simplest  InputSameDT=on
  Lookup Table PA : Lookup_n-D  NumberOfTableDimensions=1  BreakpointsForDimension1=Valve.lookupspoolPA  Table=Valve.lookupopenPA  InternalRulePriority=Speed  RndMeth=Simplest  InputSameDT=on
  Lookup Table PB : Lookup_n-D  NumberOfTableDimensions=1  BreakpointsForDimension1=Valve.lookupspoolPB  Table=Valve.lookupopenPB  InternalRulePriority=Speed  RndMeth=Simplest  InputSameDT=on
  av_AT : Outport
  av_BT : Outport  Port=2
  av_PB : Outport  Port=3
  av_PA : Outport  Port=4
  wires:
  x/1 -> Lookup Table AT/1, Lookup Table PB/1, Lookup Table BT/1, Lookup Table PA/1
  Lookup Table AT/1 -> av_AT/1
  Lookup Table PA/1 -> av_PA/1
  Lookup Table BT/1 -> av_BT/1
  Lookup Table PB/1 -> av_PB/1

== system simulink/Hydraulics/Cylinder 2/4//3 Valve/Valve Dynamics ==
  u : Inport
  Saturation1 : Saturate  UpperLimit=1  LowerLimit=-1
  Transfer Fcn1 : TransferFcn  Numerator=[(Valve_omega)^2]  Denominator=[1 2*Valve_eta*Valve_omega (Valve_omega)^2]
  Transport Delay1 : TransportDelay  DelayTime=Valve.secondorder_delay
  x : Outport
  wires:
  Transfer Fcn1/1 -> Saturation1/1
  u/1 -> Transport Delay1/1
  Saturation1/1 -> x/1
  Transport Delay1/1 -> Transfer Fcn1/1

== system simulink/Hydraulics/Cylinder 2/Cylinder/A_chamber size ==
  x : Inport
  A_Dead Vol : Constant  Value=Cyl.V0A
  A_plunger area : Gain  Gain=Cyl2.A_A
  Add1 : Sum
  V_A : Outport
  wires:
  A_Dead Vol/1 -> Add1/2
  A_plunger area/1 -> Add1/1
  x/1 -> A_plunger area/1
  Add1/1 -> V_A/1

== system simulink/Hydraulics/Cylinder 2/Cylinder/B_chamber size ==
  x : Inport
  Add2 : Sum  Inputs=-+
  Add4 : Sum
  B_Dead Vol : Constant  Value=Cyl.V0B
  B_plunger area : Gain  Gain=Cyl2.A_B
  Cyl_stroke : Constant  Value=Cyl2.xmax
  V_B : Outport
  wires:
  Add4/1 -> V_B/1
  B_Dead Vol/1 -> Add4/2
  B_plunger area/1 -> Add4/1
  Add2/1 -> B_plunger area/1
  x/1 -> Add2/1
  Cyl_stroke/1 -> Add2/2

== system simulink/Hydraulics/Cylinder 2/Cylinder/Chamber A ==
  Q_in : Inport
  " dv_A/dt" : Inport  Port=2
  " V_A" : Inport  Port=3
  " B" : Inport  Port=4
  Integrator : Integrator  InitialCondition=pinitial  AbsoluteTolerance=10
  Product : Product  Inputs=*/*  SaturateOnIntegerOverflow=on  InputSameDT=on  OutDataTypeStr=Inherit: Same as first input
  Saturation : Saturate  UpperLimit=inf  LowerLimit=0
  Sum : Sum  Inputs=+-  SaturateOnIntegerOverflow=on  InputSameDT=on  OutDataTypeStr=Inherit: Same as first input
  p_A : Outport
  wires:
  Sum/1 -> Product/1
  Q_in/1 -> Sum/1
  " B"/1 -> Product/3
  Saturation/1 -> p_A/1
  Integrator/1 -> Saturation/1
  Product/1 -> Integrator/1
  " dv_A/dt"/1 -> Sum/2
  " V_A"/1 -> Product/2

== system simulink/Hydraulics/Cylinder 2/Cylinder/Chamber B ==
  B : Inport
  V_B : Inport  Port=2
  dv_B/dt : Inport  Port=3
  Q_in : Inport  Port=4
  Integrator : Integrator  InitialCondition=pinitial  AbsoluteTolerance=10
  Product : Product  Inputs=*/*  SaturateOnIntegerOverflow=on  InputSameDT=on  OutDataTypeStr=Inherit: Same as first input
  Saturation : Saturate  UpperLimit=inf  LowerLimit=0
  Sum : Sum  Inputs=+-  SaturateOnIntegerOverflow=on  InputSameDT=on  OutDataTypeStr=Inherit: Same as first input
  p_B : Outport
  wires:
  Product/1 -> Integrator/1
  Integrator/1 -> Saturation/1
  Saturation/1 -> p_B/1
  B/1 -> Product/3
  Q_in/1 -> Sum/1
  Sum/1 -> Product/1
  dv_B/dt/1 -> Sum/2
  V_B/1 -> Product/2

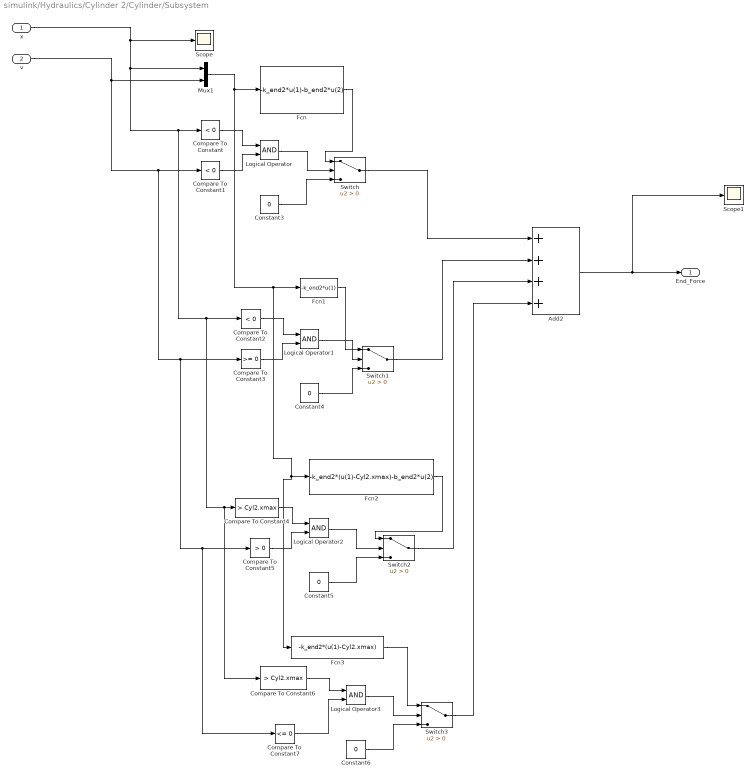
== system simulink/Hydraulics/Cylinder 2/Cylinder/Subsystem ==
  x : Inport
  v : Inport  Port=2
  Add2 : Sum  Inputs=++++
  Compare To Constant : simulink/Logic and Bit Operations/Compare To Constant  relop=<  const=0  OutDataTypeStr=boolean
  Compare To Constant1 : simulink/Logic and Bit Operations/Compare To Constant  relop=<  const=0  OutDataTypeStr=boolean
  Compare To Constant2 : simulink/Logic and Bit Operations/Compare To Constant  relop=<  const=0  OutDataTypeStr=boolean
  Compare To Constant3 : simulink/Logic and Bit Operations/Compare To Constant  relop=>=  const=0  OutDataTypeStr=boolean
  Compare To Constant4 : simulink/Logic and Bit Operations/Compare To Constant  relop=>  const=Cyl2.xmax  OutDataTypeStr=boolean
  Compare To Constant5 : simulink/Logic and Bit Operations/Compare To Constant  relop=>  const=0  OutDataTypeStr=boolean
  Compare To Constant6 : simulink/Logic and Bit Operations/Compare To Constant  relop=>  const=Cyl2.xmax  OutDataTypeStr=boolean
  Compare To Constant7 : simulink/Logic and Bit Operations/Compare To Constant  relop=<=  const=0  OutDataTypeStr=boolean
  Constant{3..6} (4 alike) : Constant  Value=0
  Fcn : Fcn  Expr=-k_end2*u(1)-b_end2*u(2)
  Fcn1 : Fcn  Expr=-k_end2*u(1)
  Fcn2 : Fcn  Expr=-k_end2*(u(1)-Cyl2.xmax)-b_end2*u(2)
  Fcn3 : Fcn  Expr=-k_end2*(u(1)-Cyl2.xmax)
  Logical Operator{,1..3} (4 alike) : Logic  AllPortsSameDT=off  OutDataTypeStr=boolean
  Mux1 : Mux  Inputs=2
  Scope : Scope
      settings: YMin=-0.16833  YMax=0.74646  SaveName=ScopeData3
  Scope1 : Scope
      settings: YMin=-1193475.02385  YMax=132608.33598  SaveName=ScopeData14
  Switch{,1..3} (4 alike) : Switch  Criteria=u2 > Threshold
  End_Force : Outport
  wires:
  Compare To Constant3/1 -> Logical Operator1/2
  Fcn1/1 -> Switch1/1
  Compare To Constant4/1 -> Logical Operator2/1
  Compare To Constant/1 -> Logical Operator/1
  Constant3/1 -> Switch/3
  Logical Operator/1 -> Switch/2
  Fcn/1 -> Switch/1
  Logical Operator1/1 -> Switch1/2
  Constant4/1 -> Switch1/3
  Constant5/1 -> Switch2/3
  Compare To Constant1/1 -> Logical Operator/2
  Compare To Constant2/1 -> Logical Operator1/1
  Switch3/1 -> Add2/4
  Mux1/1 -> Fcn/1, Fcn3/1, Fcn2/1, Fcn1/1
  Add2/1 -> Scope1/1, End_Force/1
  Switch1/1 -> Add2/2
  Compare To Constant7/1 -> Logical Operator3/2
  Logical Operator2/1 -> Switch2/2
  Switch/1 -> Add2/1
  Compare To Constant6/1 -> Logical Operator3/1
  Switch2/1 -> Add2/3
  Constant6/1 -> Switch3/3
  Compare To Constant5/1 -> Logical Operator2/2
  Fcn3/1 -> Switch3/1
  Logical Operator3/1 -> Switch3/2
  Fcn2/1 -> Switch2/1
  v/1 -> Compare To Constant7/1, Compare To Constant5/1, Compare To Constant3/1, Compare To Constant1/1, Mux1/2
  x/1 -> Scope/1, Mux1/1, Compare To Constant4/1, Compare To Constant6/1, Compare To Constant2/1, Compare To Constant/1

== system simulink/Hydraulics/Cylinder 3/4//3 Valve/Flow paths ==
  p_A : Inport
  p_B : Inport  Port=2
  p_S : Inport  Port=3
  p_T : Inport  Port=4
  av_AT : Inport  Port=5
  av_BT : Inport  Port=6
  av_PB : Inport  Port=7
  av_PA : Inport  Port=8
  Orifice AT : Subsystem  mask(Hydraulic){QN=Valve3.QN.AT, dpN=Valve3.dpN, ptr=Valve3.ptr}
      mask prompts: QN "Nominal Flow [m^3/s] :"; dpN "Nominal Pressure Difference [Pa] :"; ptr "Transition Pressure [Pa] :"
      mask help:
      | Implements numerically robust turbulent flow
      | equation. Polynomial flow equation is used
      | when abs(dp) < Transition Pressure.
      mask init:
      | K = QN/(sqrt(dpN));
      mask Help: eval('hydlibdoc(''orificedoc'')')
  Orifice BT : Subsystem  mask(Hydraulic){QN=Valve3.QN.BT, dpN=Valve3.dpN, ptr=Valve3.ptr}
      mask prompts: QN "Nominal Flow [m^3/s] :"; dpN "Nominal Pressure Difference [Pa] :"; ptr "Transition Pressure [Pa] :"
      mask help:
      | Implements numerically robust turbulent flow
      | equation. Polynomial flow equation is used
      | when abs(dp) < Transition Pressure.
      mask init:
      | K = QN/(sqrt(dpN));
      mask Help: eval('hydlibdoc(''orificedoc'')')
  Orifice PA : Subsystem  mask(Hydraulic){QN=Valve3.QN.PA, dpN=Valve3.dpN, ptr=Valve3.ptr}
      mask prompts: QN "Nominal Flow [m^3/s] :"; dpN "Nominal Pressure Difference [Pa] :"; ptr "Transition Pressure [Pa] :"
      mask help:
      | Implements numerically robust turbulent flow
      | equation. Polynomial flow equation is used
      | when abs(dp) < Transition Pressure.
      mask init:
      | K = QN/(sqrt(dpN));
      mask Help: eval('hydlibdoc(''orificedoc'')')
  Orifice PB : Subsystem  mask(Hydraulic){QN=Valve3.QN.PB, dpN=Valve3.dpN, ptr=Valve3.ptr}
      mask prompts: QN "Nominal Flow [m^3/s] :"; dpN "Nominal Pressure Difference [Pa] :"; ptr "Transition Pressure [Pa] :"
      mask help:
      | Implements numerically robust turbulent flow
      | equation. Polynomial flow equation is used
      | when abs(dp) < Transition Pressure.
      mask init:
      | K = QN/(sqrt(dpN));
      mask Help: eval('hydlibdoc(''orificedoc'')')
  Sum{,1..3} (4 alike) : Sum  Inputs=|++
  Q_A : Outport
  Q_P : Outport  Port=2
  Q_T : Outport  Port=3
  Q_B : Outport  Port=4
  wires:
  p_A/1 -> Orifice AT/1(p_A), Orifice PA/2(p_A)
  p_T/1 -> Orifice BT/1(p_T), Orifice AT/2(p_T)
  av_BT/1 -> Orifice BT/3(u)
  av_PA/1 -> Orifice PA/3(u)
  p_B/1 -> Orifice PB/1(p_B), Orifice BT/2(p_B)
  av_PB/1 -> Orifice PB/3(u)
  p_S/1 -> Orifice PB/2(p_P), Orifice PA/1(p_P)
  av_AT/1 -> Orifice AT/3(u)
  Orifice PA/2(Q_A) -> Sum/1
  Orifice AT/1(Q_A) -> Sum/2
  Orifice AT/2(Q_T) -> Sum3/1
  Orifice BT/1(Q_T) -> Sum3/2
  Orifice BT/2(Q_B) -> Sum2/1
  Orifice PB/1(Q_B) -> Sum2/2
  Orifice PA/1(Q_P) -> Sum1/1
  Orifice PB/2(Q_P) -> Sum1/2
  Sum/1 -> Q_A/1
  Sum1/1 -> Q_P/1
  Sum3/1 -> Q_T/1
  Sum2/1 -> Q_B/1

== system simulink/Hydraulics/Cylinder 3/4//3 Valve/Relative openings ==
  x : Inport
  Lookup Table AT : Lookup_n-D  NumberOfTableDimensions=1  BreakpointsForDimension1=Valve.lookupspoolAT  Table=Valve.lookupopenAT  InternalRulePriority=Speed  RndMeth=Simplest  InputSameDT=on
  Lookup Table BT : Lookup_n-D  NumberOfTableDimensions=1  BreakpointsForDimension1=Valve.lookupspoolBT  Table=Valve.lookupopenBT  InternalRulePriority=Speed  RndMeth=Simplest  InputSameDT=on
  Lookup Table PA : Lookup_n-D  NumberOfTableDimensions=1  BreakpointsForDimension1=Valve.lookupspoolPA  Table=Valve.lookupopenPA  InternalRulePriority=Speed  RndMeth=Simplest  InputSameDT=on
  Lookup Table PB : Lookup_n-D  NumberOfTableDimensions=1  BreakpointsForDimension1=Valve.lookupspoolPB  Table=Valve.lookupopenPB  InternalRulePriority=Speed  RndMeth=Simplest  InputSameDT=on
  av_AT : Outport
  av_BT : Outport  Port=2
  av_PB : Outport  Port=3
  av_PA : Outport  Port=4
  wires:
  x/1 -> Lookup Table AT/1, Lookup Table PB/1, Lookup Table BT/1, Lookup Table PA/1
  Lookup Table AT/1 -> av_AT/1
  Lookup Table PA/1 -> av_PA/1
  Lookup Table BT/1 -> av_BT/1
  Lookup Table PB/1 -> av_PB/1

== system simulink/Hydraulics/Cylinder 3/4//3 Valve/Valve Dynamics ==
  u : Inport
  Saturation1 : Saturate  UpperLimit=1  LowerLimit=-1
  Transfer Fcn1 : TransferFcn  Numerator=[(Valve_omega)^2]  Denominator=[1 2*Valve_eta*Valve_omega (Valve_omega)^2]
  Transport Delay1 : TransportDelay  DelayTime=Valve.secondorder_delay
  x : Outport
  wires:
  Transfer Fcn1/1 -> Saturation1/1
  u/1 -> Transport Delay1/1
  Saturation1/1 -> x/1
  Transport Delay1/1 -> Transfer Fcn1/1

== system simulink/Hydraulics/Cylinder 3/Cylinder/A_chamber size ==
  x : Inport
  A_Dead Vol : Constant  Value=Cyl.V0A
  A_plunger area : Gain  Gain=Cyl3.A_A
  Add1 : Sum
  V_A : Outport
  wires:
  A_Dead Vol/1 -> Add1/2
  A_plunger area/1 -> Add1/1
  x/1 -> A_plunger area/1
  Add1/1 -> V_A/1

== system simulink/Hydraulics/Cylinder 3/Cylinder/B_chamber size ==
  x : Inport
  Add2 : Sum  Inputs=-+
  Add4 : Sum
  B_Dead Vol : Constant  Value=Cyl.V0B
  B_plunger area : Gain  Gain=Cyl3.A_B
  Cyl_stroke : Constant  Value=Cyl3.xmax
  V_B : Outport
  wires:
  Add4/1 -> V_B/1
  B_Dead Vol/1 -> Add4/2
  B_plunger area/1 -> Add4/1
  Add2/1 -> B_plunger area/1
  x/1 -> Add2/1
  Cyl_stroke/1 -> Add2/2

== system simulink/Hydraulics/Cylinder 3/Cylinder/Chamber A ==
  Q_in : Inport
  " dv_A/dt" : Inport  Port=2
  " V_A" : Inport  Port=3
  " B" : Inport  Port=4
  Integrator : Integrator  InitialCondition=pinitial  AbsoluteTolerance=10
  Product : Product  Inputs=*/*  SaturateOnIntegerOverflow=on  InputSameDT=on  OutDataTypeStr=Inherit: Same as first input
  Saturation : Saturate  UpperLimit=inf  LowerLimit=0
  Sum : Sum  Inputs=+-  SaturateOnIntegerOverflow=on  InputSameDT=on  OutDataTypeStr=Inherit: Same as first input
  p_A : Outport
  wires:
  Sum/1 -> Product/1
  Q_in/1 -> Sum/1
  " B"/1 -> Product/3
  Saturation/1 -> p_A/1
  Integrator/1 -> Saturation/1
  Product/1 -> Integrator/1
  " dv_A/dt"/1 -> Sum/2
  " V_A"/1 -> Product/2

== system simulink/Hydraulics/Cylinder 3/Cylinder/Chamber B ==
  B : Inport
  V_B : Inport  Port=2
  dv_B/dt : Inport  Port=3
  Q_in : Inport  Port=4
  Integrator : Integrator  InitialCondition=pinitial  AbsoluteTolerance=10
  Product : Product  Inputs=*/*  SaturateOnIntegerOverflow=on  InputSameDT=on  OutDataTypeStr=Inherit: Same as first input
  Saturation : Saturate  UpperLimit=inf  LowerLimit=0
  Sum : Sum  Inputs=+-  SaturateOnIntegerOverflow=on  InputSameDT=on  OutDataTypeStr=Inherit: Same as first input
  p_B : Outport
  wires:
  Product/1 -> Integrator/1
  Integrator/1 -> Saturation/1
  Saturation/1 -> p_B/1
  B/1 -> Product/3
  Q_in/1 -> Sum/1
  Sum/1 -> Product/1
  dv_B/dt/1 -> Sum/2
  V_B/1 -> Product/2

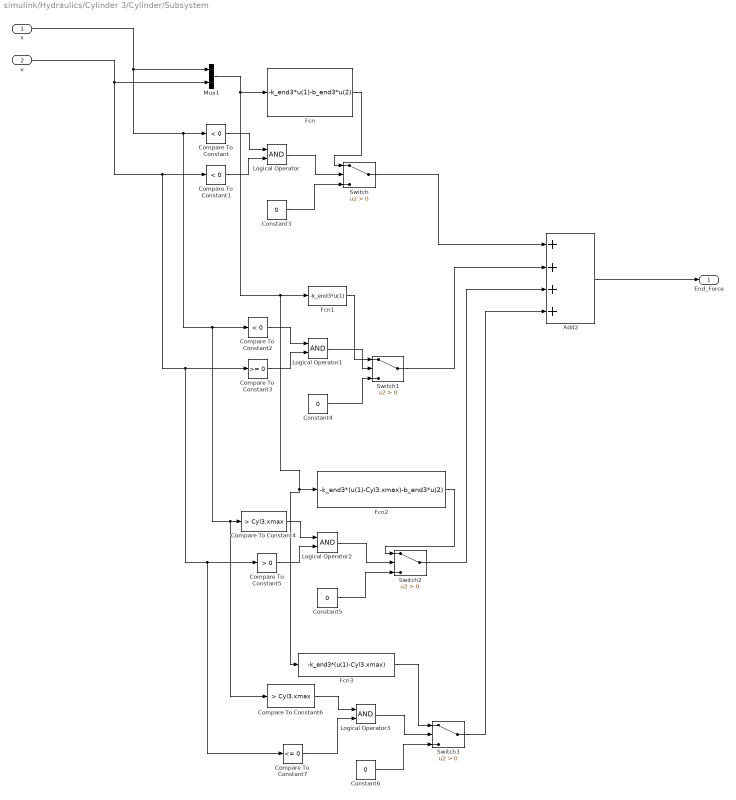
== system simulink/Hydraulics/Cylinder 3/Cylinder/Subsystem ==
  x : Inport
  v : Inport  Port=2
  Add2 : Sum  Inputs=++++
  Compare To Constant : simulink/Logic and Bit Operations/Compare To Constant  relop=<  const=0  OutDataTypeStr=boolean
  Compare To Constant1 : simulink/Logic and Bit Operations/Compare To Constant  relop=<  const=0  OutDataTypeStr=boolean
  Compare To Constant2 : simulink/Logic and Bit Operations/Compare To Constant  relop=<  const=0  OutDataTypeStr=boolean
  Compare To Constant3 : simulink/Logic and Bit Operations/Compare To Constant  relop=>=  const=0  OutDataTypeStr=boolean
  Compare To Constant4 : simulink/Logic and Bit Operations/Compare To Constant  relop=>  const=Cyl3.xmax  OutDataTypeStr=boolean
  Compare To Constant5 : simulink/Logic and Bit Operations/Compare To Constant  relop=>  const=0  OutDataTypeStr=boolean
  Compare To Constant6 : simulink/Logic and Bit Operations/Compare To Constant  relop=>  const=Cyl3.xmax  OutDataTypeStr=boolean
  Compare To Constant7 : simulink/Logic and Bit Operations/Compare To Constant  relop=<=  const=0  OutDataTypeStr=boolean
  Constant{3..6} (4 alike) : Constant  Value=0
  Fcn : Fcn  Expr=-k_end3*u(1)-b_end3*u(2)
  Fcn1 : Fcn  Expr=-k_end3*u(1)
  Fcn2 : Fcn  Expr=-k_end3*(u(1)-Cyl3.xmax)-b_end3*u(2)
  Fcn3 : Fcn  Expr=-k_end3*(u(1)-Cyl3.xmax)
  Logical Operator{,1..3} (4 alike) : Logic  AllPortsSameDT=off  OutDataTypeStr=boolean
  Mux1 : Mux  Inputs=2
  Switch{,1..3} (4 alike) : Switch  Criteria=u2 > Threshold
  End_Force : Outport
  wires:
  Compare To Constant3/1 -> Logical Operator1/2
  Fcn1/1 -> Switch1/1
  Compare To Constant4/1 -> Logical Operator2/1
  Compare To Constant/1 -> Logical Operator/1
  Constant3/1 -> Switch/3
  Logical Operator/1 -> Switch/2
  Fcn/1 -> Switch/1
  Logical Operator1/1 -> Switch1/2
  Constant4/1 -> Switch1/3
  Constant5/1 -> Switch2/3
  Compare To Constant1/1 -> Logical Operator/2
  Compare To Constant2/1 -> Logical Operator1/1
  Switch3/1 -> Add2/4
  Mux1/1 -> Fcn/1, Fcn3/1, Fcn2/1, Fcn1/1
  Add2/1 -> End_Force/1
  Switch1/1 -> Add2/2
  Compare To Constant7/1 -> Logical Operator3/2
  Logical Operator2/1 -> Switch2/2
  Switch/1 -> Add2/1
  Compare To Constant6/1 -> Logical Operator3/1
  Switch2/1 -> Add2/3
  Constant6/1 -> Switch3/3
  Compare To Constant5/1 -> Logical Operator2/2
  Fcn3/1 -> Switch3/1
  Logical Operator3/1 -> Switch3/2
  Fcn2/1 -> Switch2/1
  v/1 -> Compare To Constant7/1, Compare To Constant5/1, Compare To Constant3/1, Compare To Constant1/1, Mux1/2
  x/1 -> Mux1/1, Compare To Constant4/1, Compare To Constant6/1, Compare To Constant2/1, Compare To Constant/1

== system simulink/Hydraulics/Cylinder 5/4//3 Valve/Flow paths ==
  p_A : Inport
  p_B : Inport  Port=2
  p_S : Inport  Port=3
  p_T : Inport  Port=4
  av_AT : Inport  Port=5
  av_BT : Inport  Port=6
  av_PB : Inport  Port=7
  av_PA : Inport  Port=8
  Orifice AT : Subsystem  mask(Hydraulic){QN=Valve4.QN.AT, dpN=Valve4.dpN, ptr=Valve4.ptr}
      mask prompts: QN "Nominal Flow [m^3/s] :"; dpN "Nominal Pressure Difference [Pa] :"; ptr "Transition Pressure [Pa] :"
      mask help:
      | Implements numerically robust turbulent flow
      | equation. Polynomial flow equation is used
      | when abs(dp) < Transition Pressure.
      mask init:
      | K = QN/(sqrt(dpN));
      mask Help: eval('hydlibdoc(''orificedoc'')')
  Orifice BT : Subsystem  mask(Hydraulic){QN=Valve4.QN.BT, dpN=Valve4.dpN, ptr=Valve4.ptr}
      mask prompts: QN "Nominal Flow [m^3/s] :"; dpN "Nominal Pressure Difference [Pa] :"; ptr "Transition Pressure [Pa] :"
      mask help:
      | Implements numerically robust turbulent flow
      | equation. Polynomial flow equation is used
      | when abs(dp) < Transition Pressure.
      mask init:
      | K = QN/(sqrt(dpN));
      mask Help: eval('hydlibdoc(''orificedoc'')')
  Orifice PA : Subsystem  mask(Hydraulic){QN=Valve4.QN.PA, dpN=Valve4.dpN, ptr=Valve4.ptr}
      mask prompts: QN "Nominal Flow [m^3/s] :"; dpN "Nominal Pressure Difference [Pa] :"; ptr "Transition Pressure [Pa] :"
      mask help:
      | Implements numerically robust turbulent flow
      | equation. Polynomial flow equation is used
      | when abs(dp) < Transition Pressure.
      mask init:
      | K = QN/(sqrt(dpN));
      mask Help: eval('hydlibdoc(''orificedoc'')')
  Orifice PB : Subsystem  mask(Hydraulic){QN=Valve4.QN.PB, dpN=Valve4.dpN, ptr=Valve4.ptr}
      mask prompts: QN "Nominal Flow [m^3/s] :"; dpN "Nominal Pressure Difference [Pa] :"; ptr "Transition Pressure [Pa] :"
      mask help:
      | Implements numerically robust turbulent flow
      | equation. Polynomial flow equation is used
      | when abs(dp) < Transition Pressure.
      mask init:
      | K = QN/(sqrt(dpN));
      mask Help: eval('hydlibdoc(''orificedoc'')')
  Sum{,1..3} (4 alike) : Sum  Inputs=|++
  Q_A : Outport
  Q_P : Outport  Port=2
  Q_T : Outport  Port=3
  Q_B : Outport  Port=4
  wires:
  Sum2/1 -> Q_B/1
  Sum3/1 -> Q_T/1
  Sum1/1 -> Q_P/1
  Sum/1 -> Q_A/1
  Orifice PB/2(Q_P) -> Sum1/2
  Orifice PA/1(Q_P) -> Sum1/1
  Orifice PB/1(Q_B) -> Sum2/2
  Orifice BT/2(Q_B) -> Sum2/1
  Orifice BT/1(Q_T) -> Sum3/2
  Orifice AT/2(Q_T) -> Sum3/1
  Orifice AT/1(Q_A) -> Sum/2
  Orifice PA/2(Q_A) -> Sum/1
  av_AT/1 -> Orifice AT/3(u)
  p_S/1 -> Orifice PA/1(p_P), Orifice PB/2(p_P)
  av_PB/1 -> Orifice PB/3(u)
  p_B/1 -> Orifice BT/2(p_B), Orifice PB/1(p_B)
  av_PA/1 -> Orifice PA/3(u)
  av_BT/1 -> Orifice BT/3(u)
  p_T/1 -> Orifice AT/2(p_T), Orifice BT/1(p_T)
  p_A/1 -> Orifice PA/2(p_A), Orifice AT/1(p_A)

== system simulink/Hydraulics/Cylinder 5/4//3 Valve/Relative openings ==
  x : Inport
  Lookup Table AT : Lookup_n-D  NumberOfTableDimensions=1  BreakpointsForDimension1=Valve.lookupspoolAT  Table=Valve.lookupopenAT  InternalRulePriority=Speed  RndMeth=Simplest  InputSameDT=on
  Lookup Table BT : Lookup_n-D  NumberOfTableDimensions=1  BreakpointsForDimension1=Valve.lookupspoolBT  Table=Valve.lookupopenBT  InternalRulePriority=Speed  RndMeth=Simplest  InputSameDT=on
  Lookup Table PA : Lookup_n-D  NumberOfTableDimensions=1  BreakpointsForDimension1=Valve.lookupspoolPA  Table=Valve.lookupopenPA  InternalRulePriority=Speed  RndMeth=Simplest  InputSameDT=on
  Lookup Table PB : Lookup_n-D  NumberOfTableDimensions=1  BreakpointsForDimension1=Valve.lookupspoolPB  Table=Valve.lookupopenPB  InternalRulePriority=Speed  RndMeth=Simplest  InputSameDT=on
  av_AT : Outport
  av_BT : Outport  Port=2
  av_PB : Outport  Port=3
  av_PA : Outport  Port=4
  wires:
  Lookup Table PB/1 -> av_PB/1
  Lookup Table BT/1 -> av_BT/1
  Lookup Table PA/1 -> av_PA/1
  Lookup Table AT/1 -> av_AT/1
  x/1 -> Lookup Table PA/1, Lookup Table BT/1, Lookup Table PB/1, Lookup Table AT/1

== system simulink/Hydraulics/Cylinder 5/4//3 Valve/Valve Dynamics ==
  u : Inport
  Saturation1 : Saturate  UpperLimit=1  LowerLimit=-1
  Transfer Fcn1 : TransferFcn  Numerator=[(Valve_omega)^2]  Denominator=[1 2*Valve_eta*Valve_omega (Valve_omega)^2]
  Transport Delay1 : TransportDelay  DelayTime=Valve.secondorder_delay
  x : Outport
  wires:
  Transport Delay1/1 -> Transfer Fcn1/1
  Saturation1/1 -> x/1
  u/1 -> Transport Delay1/1
  Transfer Fcn1/1 -> Saturation1/1

== system simulink/Hydraulics/Cylinder 5/Cylinder/A_chamber size ==
  x : Inport
  A_Dead Vol : Constant  Value=Cyl.V0A
  A_plunger area : Gain  Gain=Cyl4.A_A
  Add1 : Sum
  V_A : Outport
  wires:
  Add1/1 -> V_A/1
  x/1 -> A_plunger area/1
  A_plunger area/1 -> Add1/1
  A_Dead Vol/1 -> Add1/2

== system simulink/Hydraulics/Cylinder 5/Cylinder/B_chamber size ==
  x : Inport
  Add2 : Sum  Inputs=-+
  Add4 : Sum
  B_Dead Vol : Constant  Value=Cyl.V0B
  B_plunger area : Gain  Gain=Cyl4.A_B
  Cyl_stroke : Constant  Value=Cyl4.xmax
  V_B : Outport
  wires:
  Cyl_stroke/1 -> Add2/2
  x/1 -> Add2/1
  Add2/1 -> B_plunger area/1
  B_plunger area/1 -> Add4/1
  B_Dead Vol/1 -> Add4/2
  Add4/1 -> V_B/1
